simulink model "SSB_Modul_Demodu"  (R2023a)
settings: Solver=VariableStepAuto  StartTime=0.0  StopTime=1  RelTol=1e-3
libraries: dspfdesign x2
settings Model: Creator=Pedro  LastModifiedBy=Pedro

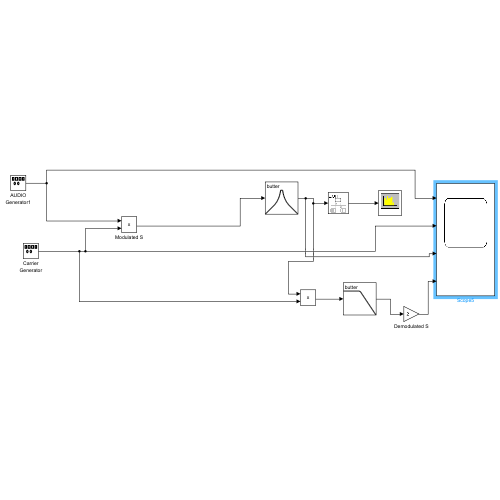
[thumbnail: Simulink's stored preview of the top-level diagram]
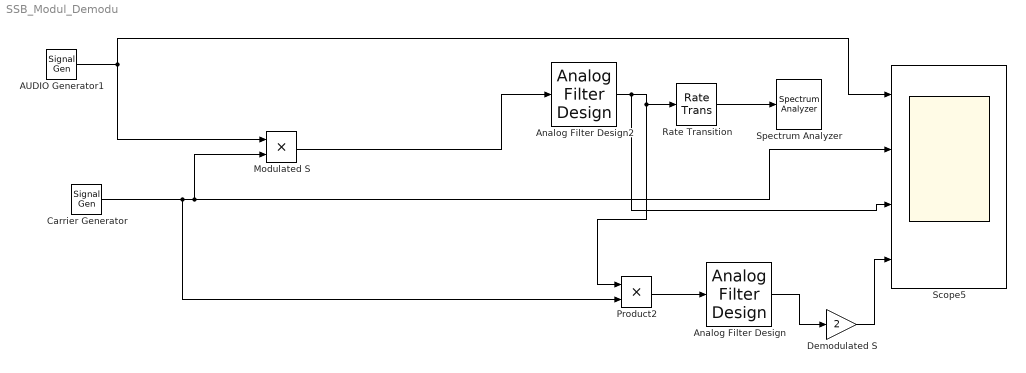
== system SSB_Modul_Demodu ==
  AUDIO Generator1 : SignalGenerator  Amplitude=1.5  Frequency=20  VectorParams1D=off
  Analog Filter Design : dspfdesign/Analog Filter Design  method=Butterworth  filttype=Lowpass  N=8  Wlo=2*pi*90  Whi=2*pi*1000  Rp=2  Rs=40
  Analog Filter Design2 : dspfdesign/Analog Filter Design  method=Butterworth  filttype=Bandpass  N=8  Wlo=2*pi*80  Whi=2*pi*100  Rp=2  Rs=40
  Carrier Generator : SignalGenerator  Frequency=110
  Demodulated S : Gain  Gain=2
  Modulated S : Product
  Product2 : Product
  Rate Transition : RateTransition  OutPortSampleTime=0.0001
  Scope5 : Scope  NumInputPorts=4
  Spectrum Analyzer : SpectrumAnalyzer  WindowPosition=[1.000000,41.000000,1280.000000,657.000000,]  ScopeFrameLocation=window  Method=Welch  SampleRate=44.1e3  PlotAsTwoSidedSpectrum=off  StartFrequency=20  StopFrequency=20e3  SpectrumUnits=Watts  YLimits=[-0.01281711,0.11535398]  SelectedToolstripTab=spectrumAnalyzerToolstrip.measurementsTab
  wires:
  Rate Transition/1 -> Spectrum Analyzer/1
  Analog Filter Design2/1 -> Scope5/3, Product2/1, Rate Transition/1
  AUDIO Generator1/1 -> Scope5/1, Modulated S/1
  Carrier Generator/1 -> Scope5/2, Modulated S/2, Product2/2
  Modulated S/1 -> Analog Filter Design2/1
  Product2/1 -> Analog Filter Design/1
  Analog Filter Design/1 -> Demodulated S/1
  Demodulated S/1 -> Scope5/4
